simulink model "cruiseControlSimulink"  (R2015b)
settings: Solver=ode45  StartTime=0.0  StopTime=10.0  RelTol=1e-3
undefined symbols (not defined in the file): kI, kp
settings Model: Creator=Rane  LastModifiedBy=rane
settings DataIOCC: SaveFormat=Array
settings DebuggingCC: SolverPrmCheckMsg=warning
settings HardwareCC: ProdBitPerPointer=32  ProdLargestAtomicFloat=None  ProdIntDivRoundTo=Undefined  ProdEndianess=Unspecified  ProdWordSize=32  ProdHWDeviceType=32-bit Generic
settings GRTTargetCC: GeneratePreprocessorConditionals=Disable all
settings ConfigComp: CovModelRefEnable=Off  CovSFcnEnable=off

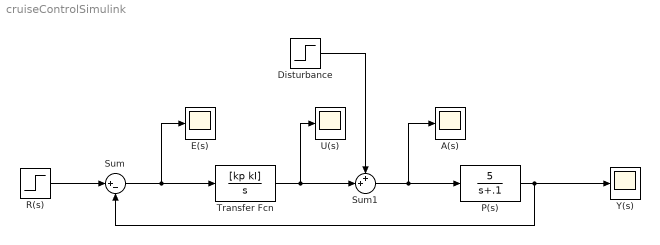
== system cruiseControlSimulink ==
  A(s) : Scope
  Disturbance : Step  After=0  SampleTime=0
  E(s) : Scope
  P(s) : TransferFcn  Numerator=[5]  Denominator=[1 .1]
  R(s) : Step  SampleTime=0
  Sum : Sum  Inputs=|+-
  Sum1 : Sum  Inputs=++|
  Transfer Fcn : TransferFcn  Numerator=[kp kI]  Denominator=[1 0]
  U(s) : Scope
  Y(s) : Scope
  wires:
  Sum1/1 -> A(s)/1, P(s)/1
  P(s)/1 -> Y(s)/1, Sum/2
  R(s)/1 -> Sum/1
  Disturbance/1 -> Sum1/1
  Transfer Fcn/1 -> Sum1/2, U(s)/1
  Sum/1 -> E(s)/1, Transfer Fcn/1
